simulink library "sm_mining_loader_lib"  (R2026a)
settings: Solver=VariableStepAuto
undefined symbols (not defined in the file): FL, FR, Init, LL, LR, Maneuver, minMachParams, motGradParams, RL, RR, simscape, SL, SR, T, X, Y, Z
libraries: sm_lib x130, nesl_utility x77, fl_lib x36, sdl_lib x11, simulink x4, $bdroot x3, sm_vehicle_utilities_lib x2, simulink_extras x2, statsLibrary x1, grid_element x1, Maneuver_Get_Pose x1
(part 2 of 6)

== system sm_mining_loader_lib/Mining Loader/Vehicle/Camera Frames F ==
  Cam Ref Ctr : sm_lib/Frames and Transforms/Reference Frame
  Cam Ref FL : sm_lib/Frames and Transforms/Reference Frame
  Cam Ref FR : sm_lib/Frames and Transforms/Reference Frame
  Cam Ref Left : sm_lib/Frames and Transforms/Reference Frame
  Cam Ref Right : sm_lib/Frames and Transforms/Reference Frame
  Cam Ref Top Down : sm_lib/Frames and Transforms/Reference Frame
  Cam Ref Top Rear Fwd : sm_lib/Frames and Transforms/Reference Frame
  Transform Ctr : sm_lib/Frames and Transforms/Rigid Transform  RotationMethod=None  FollAlignAxisA=+X  BaseAlignAxisA=+Y  FollAlignAxisB=+Y  BaseAlignAxisB=+Z  RotationStandardAxis=+Z  RotationAngle=0  RotationAngleUnits=deg  RotationArbitraryAxis=[0 0 1]  RotationSequenceAxes=FollowerAxes  RotationSequence=XYX  RotationSequenceAngles=[0 0 0]  RotationSequenceAnglesUnits=deg  RotationMatrix=[1 0 0;0 1 0;0 0 1]  Quaternion=[1 0 0 0]  TranslationMethod=StandardAxis  TranslationCartesianOffset=[0 0 0]  TranslationCartesianOffsetUnits=m  TranslationStandardAxis=+Z  TranslationStandardOffset=2  TranslationStandardOffsetUnits=m  TranslationROffset=0  TranslationROffsetUnits=m  TranslationThetaOffset=0  TranslationThetaOffsetUnits=deg  TranslationZOffset=0  TranslationZOffsetUnits=m
  Transform FL : sm_lib/Frames and Transforms/Rigid Transform  RotationMethod=None  FollAlignAxisA=+X  BaseAlignAxisA=+Y  FollAlignAxisB=+Y  BaseAlignAxisB=+Z  RotationStandardAxis=+Z  RotationAngle=0  RotationAngleUnits=deg  RotationArbitraryAxis=[0 0 1]  RotationSequenceAxes=FollowerAxes  RotationSequence=XYX  RotationSequenceAngles=[0 0 0]  RotationSequenceAnglesUnits=deg  RotationMatrix=[1 0 0;0 1 0;0 0 1]  Quaternion=[1 0 0 0]  TranslationMethod=Cartesian  TranslationCartesianOffset=[9 5 2]  TranslationCartesianOffsetUnits=m  TranslationStandardAxis=+Z  TranslationStandardOffset=2  TranslationStandardOffsetUnits=m  TranslationROffset=0  TranslationROffsetUnits=m  TranslationThetaOffset=0  TranslationThetaOffsetUnits=deg  TranslationZOffset=0  TranslationZOffsetUnits=m
  Transform FR : sm_lib/Frames and Transforms/Rigid Transform  RotationMethod=None  FollAlignAxisA=+X  BaseAlignAxisA=+Y  FollAlignAxisB=+Y  BaseAlignAxisB=+Z  RotationStandardAxis=+Z  RotationAngle=0  RotationAngleUnits=deg  RotationArbitraryAxis=[0 0 1]  RotationSequenceAxes=FollowerAxes  RotationSequence=XYX  RotationSequenceAngles=[0 0 0]  RotationSequenceAnglesUnits=deg  RotationMatrix=[1 0 0;0 1 0;0 0 1]  Quaternion=[1 0 0 0]  TranslationMethod=Cartesian  TranslationCartesianOffset=[9 -5 2]  TranslationCartesianOffsetUnits=m  TranslationStandardAxis=+Z  TranslationStandardOffset=2  TranslationStandardOffsetUnits=m  TranslationROffset=0  TranslationROffsetUnits=m  TranslationThetaOffset=0  TranslationThetaOffsetUnits=deg  TranslationZOffset=0  TranslationZOffsetUnits=m
  Transform Left : sm_lib/Frames and Transforms/Rigid Transform  RotationMethod=None  FollAlignAxisA=+X  BaseAlignAxisA=+Y  FollAlignAxisB=+Y  BaseAlignAxisB=+Z  RotationStandardAxis=+Z  RotationAngle=0  RotationAngleUnits=deg  RotationArbitraryAxis=[0 0 1]  RotationSequenceAxes=FollowerAxes  RotationSequence=XYX  RotationSequenceAngles=[0 0 0]  RotationSequenceAnglesUnits=deg  RotationMatrix=[1 0 0;0 1 0;0 0 1]  Quaternion=[1 0 0 0]  TranslationMethod=Cartesian  TranslationCartesianOffset=[-2 -9 0]  TranslationCartesianOffsetUnits=m  TranslationStandardAxis=+Z  TranslationStandardOffset=2  TranslationStandardOffsetUnits=m  TranslationROffset=0  TranslationROffsetUnits=m  TranslationThetaOffset=0  TranslationThetaOffsetUnits=deg  TranslationZOffset=0  TranslationZOffsetUnits=m
  Transform Right : sm_lib/Frames and Transforms/Rigid Transform  RotationMethod=None  FollAlignAxisA=+X  BaseAlignAxisA=+Y  FollAlignAxisB=+Y  BaseAlignAxisB=+Z  RotationStandardAxis=+Z  RotationAngle=0  RotationAngleUnits=deg  RotationArbitraryAxis=[0 0 1]  RotationSequenceAxes=FollowerAxes  RotationSequence=XYX  RotationSequenceAngles=[0 0 0]  RotationSequenceAnglesUnits=deg  RotationMatrix=[1 0 0;0 1 0;0 0 1]  Quaternion=[1 0 0 0]  TranslationMethod=Cartesian  TranslationCartesianOffset=[-2 9 0]  TranslationCartesianOffsetUnits=m  TranslationStandardAxis=+Z  TranslationStandardOffset=2  TranslationStandardOffsetUnits=m  TranslationROffset=0  TranslationROffsetUnits=m  TranslationThetaOffset=0  TranslationThetaOffsetUnits=deg  TranslationZOffset=0  TranslationZOffsetUnits=m
  Transform Top : sm_lib/Frames and Transforms/Rigid Transform  RotationMethod=None  FollAlignAxisA=+X  BaseAlignAxisA=+Y  FollAlignAxisB=+Y  BaseAlignAxisB=+Z  RotationStandardAxis=+Z  RotationAngle=0  RotationAngleUnits=deg  RotationArbitraryAxis=[0 0 1]  RotationSequenceAxes=FollowerAxes  RotationSequence=XYX  RotationSequenceAngles=[0 0 0]  RotationSequenceAnglesUnits=deg  RotationMatrix=[1 0 0;0 1 0;0 0 1]  Quaternion=[1 0 0 0]  TranslationMethod=Cartesian  TranslationCartesianOffset=[-2 0 13]  TranslationCartesianOffsetUnits=m  TranslationStandardAxis=+Z  TranslationStandardOffset=10  TranslationStandardOffsetUnits=m  TranslationROffset=0  TranslationROffsetUnits=m  TranslationThetaOffset=0  TranslationThetaOffsetUnits=deg  TranslationZOffset=0  TranslationZOffsetUnits=m
  Transform Top Rear Fwd : sm_lib/Frames and Transforms/Rigid Transform  RotationMethod=None  FollAlignAxisA=+X  BaseAlignAxisA=+Y  FollAlignAxisB=+Y  BaseAlignAxisB=+Z  RotationStandardAxis=+Z  RotationAngle=0  RotationAngleUnits=deg  RotationArbitraryAxis=[0 0 1]  RotationSequenceAxes=FollowerAxes  RotationSequence=XYX  RotationSequenceAngles=[0 0 0]  RotationSequenceAnglesUnits=deg  RotationMatrix=[1 0 0;0 1 0;0 0 1]  Quaternion=[1 0 0 0]  TranslationMethod=Cartesian  TranslationCartesianOffset=[-4 0 1]  TranslationCartesianOffsetUnits=m  TranslationStandardAxis=+Z  TranslationStandardOffset=2  TranslationStandardOffsetUnits=m  TranslationROffset=0  TranslationROffsetUnits=m  TranslationThetaOffset=0  TranslationThetaOffsetUnits=deg  TranslationZOffset=0  TranslationZOffsetUnits=m
  R : PMIOPort  Side=Left
  connections:
  Cam Ref FL/RConn1 -- Transform FL/RConn1
  Cam Ref FR/RConn1 -- Transform FR/RConn1
  Transform Ctr/LConn1 -- R/RConn1
  Transform Top/LConn1 -- Transform Left/LConn1 -- Transform Right/LConn1 -- Cam Ref Ctr/RConn1 -- Transform FL/LConn1 -- Transform Top Rear Fwd/LConn1 -- Transform Ctr/RConn1 -- Transform FR/LConn1
  Cam Ref Right/RConn1 -- Transform Right/RConn1
  Cam Ref Left/RConn1 -- Transform Left/RConn1
  Cam Ref Top Down/RConn1 -- Transform Top/RConn1
  Cam Ref Top Rear Fwd/RConn1 -- Transform Top Rear Fwd/RConn1

== system sm_mining_loader_lib/Mining Loader/Vehicle/Camera Frames R ==
  Cam Ref Ctr : sm_lib/Frames and Transforms/Reference Frame
  Cam Ref LR : sm_lib/Frames and Transforms/Reference Frame
  Cam Ref Left : sm_lib/Frames and Transforms/Reference Frame
  Cam Ref RR : sm_lib/Frames and Transforms/Reference Frame
  Cam Ref Right : sm_lib/Frames and Transforms/Reference Frame
  Cam Ref Top Down : sm_lib/Frames and Transforms/Reference Frame
  Cam Ref Top Rear Fwd : sm_lib/Frames and Transforms/Reference Frame
  Transform Ctr : sm_lib/Frames and Transforms/Rigid Transform  RotationMethod=None  FollAlignAxisA=+X  BaseAlignAxisA=+Y  FollAlignAxisB=+Y  BaseAlignAxisB=+Z  RotationStandardAxis=+Z  RotationAngle=0  RotationAngleUnits=deg  RotationArbitraryAxis=[0 0 1]  RotationSequenceAxes=FollowerAxes  RotationSequence=XYX  RotationSequenceAngles=[0 0 0]  RotationSequenceAnglesUnits=deg  RotationMatrix=[1 0 0;0 1 0;0 0 1]  Quaternion=[1 0 0 0]  TranslationMethod=StandardAxis  TranslationCartesianOffset=[0 0 0]  TranslationCartesianOffsetUnits=m  TranslationStandardAxis=+Z  TranslationStandardOffset=2  TranslationStandardOffsetUnits=m  TranslationROffset=0  TranslationROffsetUnits=m  TranslationThetaOffset=0  TranslationThetaOffsetUnits=deg  TranslationZOffset=0  TranslationZOffsetUnits=m
  Transform LR : sm_lib/Frames and Transforms/Rigid Transform  RotationMethod=None  FollAlignAxisA=+X  BaseAlignAxisA=+Y  FollAlignAxisB=+Y  BaseAlignAxisB=+Z  RotationStandardAxis=+Z  RotationAngle=0  RotationAngleUnits=deg  RotationArbitraryAxis=[0 0 1]  RotationSequenceAxes=FollowerAxes  RotationSequence=XYX  RotationSequenceAngles=[0 0 0]  RotationSequenceAnglesUnits=deg  RotationMatrix=[1 0 0;0 1 0;0 0 1]  Quaternion=[1 0 0 0]  TranslationMethod=Cartesian  TranslationCartesianOffset=[-8 -5 2]  TranslationCartesianOffsetUnits=m  TranslationStandardAxis=+Z  TranslationStandardOffset=2  TranslationStandardOffsetUnits=m  TranslationROffset=0  TranslationROffsetUnits=m  TranslationThetaOffset=0  TranslationThetaOffsetUnits=deg  TranslationZOffset=0  TranslationZOffsetUnits=m
  Transform Left : sm_lib/Frames and Transforms/Rigid Transform  RotationMethod=None  FollAlignAxisA=+X  BaseAlignAxisA=+Y  FollAlignAxisB=+Y  BaseAlignAxisB=+Z  RotationStandardAxis=+Z  RotationAngle=0  RotationAngleUnits=deg  RotationArbitraryAxis=[0 0 1]  RotationSequenceAxes=FollowerAxes  RotationSequence=XYX  RotationSequenceAngles=[0 0 0]  RotationSequenceAnglesUnits=deg  RotationMatrix=[1 0 0;0 1 0;0 0 1]  Quaternion=[1 0 0 0]  TranslationMethod=Cartesian  TranslationCartesianOffset=[1.85 -9 0]  TranslationCartesianOffsetUnits=m  TranslationStandardAxis=+Z  TranslationStandardOffset=2  TranslationStandardOffsetUnits=m  TranslationROffset=0  TranslationROffsetUnits=m  TranslationThetaOffset=0  TranslationThetaOffsetUnits=deg  TranslationZOffset=0  TranslationZOffsetUnits=m
  Transform RR : sm_lib/Frames and Transforms/Rigid Transform  RotationMethod=None  FollAlignAxisA=+X  BaseAlignAxisA=+Y  FollAlignAxisB=+Y  BaseAlignAxisB=+Z  RotationStandardAxis=+Z  RotationAngle=0  RotationAngleUnits=deg  RotationArbitraryAxis=[0 0 1]  RotationSequenceAxes=FollowerAxes  RotationSequence=XYX  RotationSequenceAngles=[0 0 0]  RotationSequenceAnglesUnits=deg  RotationMatrix=[1 0 0;0 1 0;0 0 1]  Quaternion=[1 0 0 0]  TranslationMethod=Cartesian  TranslationCartesianOffset=[-8 5 2]  TranslationCartesianOffsetUnits=m  TranslationStandardAxis=+Z  TranslationStandardOffset=2  TranslationStandardOffsetUnits=m  TranslationROffset=0  TranslationROffsetUnits=m  TranslationThetaOffset=0  TranslationThetaOffsetUnits=deg  TranslationZOffset=0  TranslationZOffsetUnits=m
  Transform Right : sm_lib/Frames and Transforms/Rigid Transform  RotationMethod=None  FollAlignAxisA=+X  BaseAlignAxisA=+Y  FollAlignAxisB=+Y  BaseAlignAxisB=+Z  RotationStandardAxis=+Z  RotationAngle=0  RotationAngleUnits=deg  RotationArbitraryAxis=[0 0 1]  RotationSequenceAxes=FollowerAxes  RotationSequence=XYX  RotationSequenceAngles=[0 0 0]  RotationSequenceAnglesUnits=deg  RotationMatrix=[1 0 0;0 1 0;0 0 1]  Quaternion=[1 0 0 0]  TranslationMethod=Cartesian  TranslationCartesianOffset=[1.85 9 0]  TranslationCartesianOffsetUnits=m  TranslationStandardAxis=+Z  TranslationStandardOffset=2  TranslationStandardOffsetUnits=m  TranslationROffset=0  TranslationROffsetUnits=m  TranslationThetaOffset=0  TranslationThetaOffsetUnits=deg  TranslationZOffset=0  TranslationZOffsetUnits=m
  Transform Top : sm_lib/Frames and Transforms/Rigid Transform  RotationMethod=None  FollAlignAxisA=+X  BaseAlignAxisA=+Y  FollAlignAxisB=+Y  BaseAlignAxisB=+Z  RotationStandardAxis=+Z  RotationAngle=0  RotationAngleUnits=deg  RotationArbitraryAxis=[0 0 1]  RotationSequenceAxes=FollowerAxes  RotationSequence=XYX  RotationSequenceAngles=[0 0 0]  RotationSequenceAnglesUnits=deg  RotationMatrix=[1 0 0;0 1 0;0 0 1]  Quaternion=[1 0 0 0]  TranslationMethod=Cartesian  TranslationCartesianOffset=[1.85 0 13]  TranslationCartesianOffsetUnits=m  TranslationStandardAxis=+Z  TranslationStandardOffset=10  TranslationStandardOffsetUnits=m  TranslationROffset=0  TranslationROffsetUnits=m  TranslationThetaOffset=0  TranslationThetaOffsetUnits=deg  TranslationZOffset=0  TranslationZOffsetUnits=m
  Transform Top Rear Fwd : sm_lib/Frames and Transforms/Rigid Transform  RotationMethod=None  FollAlignAxisA=+X  BaseAlignAxisA=+Y  FollAlignAxisB=+Y  BaseAlignAxisB=+Z  RotationStandardAxis=+Z  RotationAngle=0  RotationAngleUnits=deg  RotationArbitraryAxis=[0 0 1]  RotationSequenceAxes=FollowerAxes  RotationSequence=XYX  RotationSequenceAngles=[0 0 0]  RotationSequenceAnglesUnits=deg  RotationMatrix=[1 0 0;0 1 0;0 0 1]  Quaternion=[1 0 0 0]  TranslationMethod=Cartesian  TranslationCartesianOffset=[-0.15 0 1]  TranslationCartesianOffsetUnits=m  TranslationStandardAxis=+Z  TranslationStandardOffset=2  TranslationStandardOffsetUnits=m  TranslationROffset=0  TranslationROffsetUnits=m  TranslationThetaOffset=0  TranslationThetaOffsetUnits=deg  TranslationZOffset=0  TranslationZOffsetUnits=m
  R : PMIOPort  Side=Left
  connections:
  Transform Top Rear Fwd/LConn1 -- Transform Ctr/RConn1 -- Transform RR/LConn1 -- Transform LR/LConn1 -- Cam Ref Ctr/RConn1 -- Transform Right/LConn1 -- Transform Top/LConn1 -- Transform Left/LConn1
  Transform Ctr/LConn1 -- R/RConn1
  Cam Ref LR/RConn1 -- Transform LR/RConn1
  Cam Ref RR/RConn1 -- Transform RR/RConn1
  Cam Ref Top Rear Fwd/RConn1 -- Transform Top Rear Fwd/RConn1
  Cam Ref Right/RConn1 -- Transform Right/RConn1
  Cam Ref Left/RConn1 -- Transform Left/RConn1
  Cam Ref Top Down/RConn1 -- Transform Top/RConn1

== system sm_mining_loader_lib/Mining Loader/Vehicle/Chassis ==
  Housing : Subsystem
      mask Display: image('sm_mining_loader_chassis_housing_IMAGE.png')
  Revolute Whl RL : Subsystem
  Revolute Whl RR : Subsystem
  Whl RL : Subsystem
      mask Display: image('sm_mining_loader_wheel_IMAGE.png')
  Whl RR : Subsystem
      mask Display: image('sm_mining_loader_wheel_IMAGE.png')
  Ref : PMIOPort  Side=Left
  Ground : PMIOPort  Port=2  Side=Left
  Hinge : PMIOPort  Port=3  Side=Right
  StrL : PMIOPort  Port=4  Side=Right
  StrR : PMIOPort  Port=5  Side=Right
  LR : PMIOPort  Port=6  Side=Right
  RR : PMIOPort  Port=7  Side=Right
  Out Bus Element : Outport  PortName=m  Element=WhlRL
  Out Bus Element1 : Outport  PortName=m  Element=WhlRR
  Out Bus Element2 : Outport  PortName=m  Element=TireRL
  Out Bus Element3 : Outport  PortName=m  Element=TireRR
  wires:
  Revolute Whl RR/1(m) -> Out Bus Element1/1
  Revolute Whl RL/1(m) -> Out Bus Element/1
  Whl RL/1(m) -> Out Bus Element2/1
  Whl RR/1(m) -> Out Bus Element3/1
  connections:
  Ground/RConn1 -- Whl RL/RConn1 -- Whl RR/RConn1
  RR/RConn1 -- Revolute Whl RR/LConn1
  Whl RR/LConn1 -- Revolute Whl RR/LConn2
  Revolute Whl RL/LConn1 -- LR/RConn1
  Whl RL/LConn1 -- Revolute Whl RL/LConn2
  Housing/LConn3 -- Ref/RConn1
  StrR/RConn1 -- Housing/LConn4
  StrL/RConn1 -- Housing/LConn1
  Housing/LConn2 -- Hinge/RConn1
  Revolute Whl RL/RConn1 -- Housing/RConn1
  Revolute Whl RR/RConn1 -- Housing/RConn2

== system sm_mining_loader_lib/Mining Loader/Vehicle/Frame ==
  Body Sensor : sm_vehicle_utilities_lib/Body Sensor  offset_body_sensor=[0 0 0]
  Housing : Subsystem
      settings: PortSchema="{\"entries\":[{\"content\":{\"sides\":[{\"content\":{\"connectorIds\":[\"LConn1\",\"LConn2\",\"LConn3\",\"LConn4\"]},\"type\":\"ConnectorPlacement.EquallySpacedRectSide\",\"uuid\":\"fdb8be9a-7bb9-4005-a3a7-01384b0c122c\"},{\"content\":{\"connectorIds\":[\"RConn1\",\"RConn2\",\"RConn3\",\"RConn4\"],\"side\":\"RIGHT\"},\"type\":\"ConnectorPlacement.EquallySpacedRectSide\",\"uuid\":\"1ae00c9e-27b3-4807-843a-3ea8306620e4\"},{\"content\":{\"side\":\"TOP\"},\"type\":\"ConnectorPlacement.EquallySpacedRectSide\",\"uuid\":\"0a0d877e-6f75-4a01-a1db-7b7603a65aa1\"},{\"content\":{\"connectorIds\":[\"RConn5\"],\"side\":\"BOTTOM\"},\"type\":\"ConnectorPlacement.EquallySpacedRectSide\",\"uuid\":\"108f17e2-93b2-4dab-87d6-e955d5a596de\"}]},\"type\":\"ConnectorPlacement.EquallySpacedConnector\",\"uuid\":\"ae288347-5c86-4488-a1cc-f8f672d51556\"}],\"packageUris\":[\"http://schema.mathworks.com/mf0/Connector/R2020b\"],\"version\":\"1.0\"}"
      mask Display: image('sm_mining_loader_frame_housing_IMAGE.png')
  Revolute Whl FL : Subsystem
  Revolute Whl FR : Subsystem
  Whl FL : Subsystem
      mask Display: image('sm_mining_loader_wheel_IMAGE.png')
  Whl FR : Subsystem
      mask Display: image('sm_mining_loader_wheel_IMAGE.png')
  Hinge : PMIOPort  Side=Left
  StrL : PMIOPort  Port=2  Side=Left
  StrR : PMIOPort  Port=3  Side=Left
  FR : PMIOPort  Port=4  Side=Left
  FL : PMIOPort  Port=5  Side=Left
  LiftL : PMIOPort  Port=6  Side=Right
  LiftR : PMIOPort  Port=7  Side=Right
  Boom : PMIOPort  Port=8  Side=Right
  Ground : PMIOPort  Port=9  Side=Right
  Ref : PMIOPort  Port=10  Side=Right
  Out Bus Element : Outport  PortName=m  Element=WhlFL
  Out Bus Element1 : Outport  PortName=m  Element=WhlFR
  Out Bus Element2 : Outport  PortName=m  Element=Body
  Out Bus Element3 : Outport  PortName=m  Element=TireFL
  Out Bus Element4 : Outport  PortName=m  Element=TireFR
  wires:
  Revolute Whl FL/1(m) -> Out Bus Element/1
  Revolute Whl FR/1(m) -> Out Bus Element1/1
  Body Sensor/1 -> Out Bus Element2/1
  Whl FL/1(m) -> Out Bus Element3/1
  Whl FR/1(m) -> Out Bus Element4/1
  connections:
  Ground/RConn1 -- Whl FL/RConn1 -- Whl FR/RConn1
  FL/RConn1 -- Revolute Whl FL/LConn1
  Whl FL/LConn1 -- Revolute Whl FL/LConn2
  FR/RConn1 -- Revolute Whl FR/LConn1
  Whl FR/LConn1 -- Revolute Whl FR/LConn2
  Body Sensor/LConn1 -- Housing/LConn4 -- Ref/RConn1
  Revolute Whl FL/RConn1 -- Housing/LConn1
  Revolute Whl FR/RConn1 -- Housing/RConn1
  StrL/RConn1 -- Housing/LConn2
  Housing/RConn5 -- Hinge/RConn1
  StrR/RConn1 -- Housing/RConn2
  Boom/RConn1 -- Housing/RConn4
  LiftL/RConn1 -- Housing/LConn3
  Housing/RConn3 -- LiftR/RConn1

== system sm_mining_loader_lib/Mining Loader/Vehicle/Implement ==
  qBucket : Inport
  qBoom : Inport  Port=2
  In Bus Element : Inport  Port=3  PortName=Load
  Boom : Subsystem
      mask Display: image('sm_mining_loader_impl_boom_IMAGE.png')
  Lift Actuators : Subsystem  mask{popup_lift_actuation=Hinge Motion}
      mask prompts: popup_lift_actuation "Lift Actuation"
      mask init:
      | bh = gcb;
      | actSetting = get_param(bh,'popup_lift_actuation');
      | switch actSetting
      |     case('Hinge Motion')
      |         labelStr = 'Hinge';
      |     case('Left Cylinder Motion')
      |         labelStr = 'Extension_L';
      |     case('Cylinder Actuation')
      |         labelStr = 'Actuation';
      | end
      | set_param([bh '/Actuation'],'LabelModeActiveChoice',labelStr)
      settings: AttributesFormatString=%<popup_lift_actuation>
      mask TypeOptions popup_lift_actuation: Hinge Motion | Left Cylinder Motion | Cylinder Actuation
      mask Display:
      | bh = gcb;
      | 
      | actSetting = get_param(bh,'popup_lift_actuation');
      | 
      | switch actSetting
      |     case('Hinge Motion')
      |         imageStr = 'sm_mining_loader_lift_hinge_motion_IMAGE.png';
      |     case('Left Cylinder Motion')
      |         imageStr = 'sm_mining_loader_lift_cyl_motion_IMAGE.png';
      |     case('Cylinder Actuation')
      |         imageStr = 'sm_mining_loader_lift_cyl_actuation_IMAGE.png';
      | end
      | image(imageStr)
  Linkage : Subsystem
      mask Display: image('sm_mining_loader_impl_bucket_IMAGE.png')
  Tilt Actuator : Subsystem  mask{popup_tilt_actuation=Hinge Motion}
      mask prompts: popup_tilt_actuation "Tilt Actuation"
      mask init:
      | bh = gcb;
      | actSetting = get_param(bh,'popup_tilt_actuation');
      | switch actSetting
      |     case('Hinge Motion')
      |         labelStr = 'Hinge';
      |     case('Cylinder Motion')
      |         labelStr = 'Extension';
      |     case('Cylinder Actuation')
      |         labelStr = 'Actuation';
      | end
      | set_param([bh '/Actuation'],'LabelModeActiveChoice',labelStr)
      settings: AttributesFormatString=%<popup_tilt_actuation>
      mask TypeOptions popup_tilt_actuation: Hinge Motion | Cylinder Motion | Cylinder Actuation
      mask Display:
      | bh = gcb;
      | 
      | actSetting = get_param(bh,'popup_tilt_actuation');
      | 
      | switch actSetting
      |     case('Hinge Motion')
      |         imageStr = 'sm_mining_loader_tilt_hinge_motion_IMAGE.png';
      |     case('Cylinder Motion')
      |         imageStr = 'sm_mining_loader_tilt_cyl_motion_IMAGE.png';
      |     case('Cylinder Actuation')
      |         imageStr = 'sm_mining_loader_tilt_cyl_actuation_IMAGE.png';
      | end
      | image(imageStr)
  LIftL : PMIOPort  Side=Left
  LiftR : PMIOPort  Port=2  Side=Left
  Frame : PMIOPort  Port=3  Side=Left
  LL : PMIOPort  Port=4  Side=Right
  LR : PMIOPort  Port=5  Side=Right
  T : PMIOPort  Port=6  Side=Right
  Lift : Outport
  Tilt : Outport  Port=2
  Bucket : Outport  Port=3
  wires:
  qBucket/1 -> Tilt Actuator/1(qBucket)
  qBoom/1 -> Lift Actuators/1(qBoom)
  Lift Actuators/1(m) -> Lift/1
  Tilt Actuator/1(m) -> Tilt/1
  Linkage/1(m) -> Bucket/1
  In Bus Element/1 -> Linkage/1(Load)
  connections:
  Lift Actuators/RConn3 -- Boom/LConn2
  Lift Actuators/RConn2 -- Boom/LConn1
  Boom/LConn3 -- Lift Actuators/RConn4
  Lift Actuators/LConn3 -- LiftR/RConn1
  Lift Actuators/LConn4 -- Frame/RConn1
  Lift Actuators/LConn2 -- LIftL/RConn1
  LR/RConn1 -- Lift Actuators/RConn1
  LL/RConn1 -- Lift Actuators/LConn1
  T/RConn1 -- Tilt Actuator/LConn1
  Boom/RConn2 -- Tilt Actuator/LConn3
  Linkage/LConn2 -- Tilt Actuator/RConn3
  Linkage/LConn3 -- Boom/RConn3
  Boom/RConn1 -- Tilt Actuator/LConn2
  Tilt Actuator/RConn2 -- Linkage/LConn1

== system sm_mining_loader_lib/Mining Loader/Vehicle/Steer ==
  qStr : Inport
  Actuation : Subsystem  Variant=on  VariantControlMode=label  LabelModeActiveChoice=Hinge
      settings: AttributesFormatString=%<LabelModeActiveChoice>
  Cylinder Left : sm_lib/Body Elements/File Solid  ExtGeomFileName=SteerCylinder.step  UnitType=FromFile  ExtGeomFileUnits=m  StepReaderType=HEX  ExportConvexHullGeometry=off  InertiaType=CalculateFromGeometry  BasedOnType=Mass  Density=1000  DensityUnits=kg/m^3  Mass=minMachParams.steerCyl.mass  MassUnits=kg  CenterOfMass=[0 0 0]  CenterOfMassUnits=m  MomentsOfInertia=[1 1 1]  MomentsOfInertiaUnits=kg*m^2  ProductsOfInertia=[0 0 0]  ProductsOfInertiaUnits=kg*m^2  GraphicType=FromGeometry  MarkerShape=Sphere  MarkerSize=10  GraphicVisPropType=SimpleVisualProperties  GraphicDiffuseColor=[0.1 0.1 0.1]  GraphicOpacity=1  GraphicSpecularColor=[0.5 0.5 0.5 1.0]  GraphicAmbientColor=[0.15 0.15 0.15 1.0]  GraphicEmissiveColor=[0.0 0.0 0.0 1.0]  GraphicShininess=75  DoExposeReferenceFrame=off  SerializedFrames=<Frames><Frame><Id>Frame1</Id><Value><Name>ToFrontChassis</Name><Origin><Source>GeometricFeature</Source><FeatureName>circular curve 12</FeatureName></Origin><PrimaryAxis><DefinedDirection>+Z</DefinedDirection><Source>ReferenceFrame</Source><SourceDirection>+Z</SourceDirection><FeatureName></FeatureName></PrimaryAxis><SecondaryAxis><DefinedDirection>+X</DefinedDirection><Source>ReferenceFrame</Source><SourceDirection>+X</SourceDirection><FeatureName></FeatureName></SecondaryAxis></Value></Frame><Frame><Id>Frame2</Id><Value><Name>ToSteerRod</Name><Origin><Source>GeometricFeature</Source><FeatureName>planar surface 2</FeatureName></Origin><PrimaryAxis><DefinedDirection>+Z</DefinedDirection><Source>ReferenceFrame</Source><SourceDirection>-Y</SourceDirection><FeatureName></FeatureName></PrimaryAxis><SecondaryAxis><DefinedDirection>+X</DefinedDirection><Source>ReferenceFrame</Source><SourceDirection>+X</SourceDirection><FeatureName></FeatureName></SecondaryAxis></Value></Frame></Frames>
  Cylinder Right : sm_lib/Body Elements/File Solid  ExtGeomFileName=SteerCylinder.step  UnitType=FromFile  ExtGeomFileUnits=m  StepReaderType=HEX  ExportConvexHullGeometry=off  InertiaType=CalculateFromGeometry  BasedOnType=Mass  Density=1000  DensityUnits=kg/m^3  Mass=minMachParams.steerCyl.mass  MassUnits=kg  CenterOfMass=[0 0 0]  CenterOfMassUnits=m  MomentsOfInertia=[1 1 1]  MomentsOfInertiaUnits=kg*m^2  ProductsOfInertia=[0 0 0]  ProductsOfInertiaUnits=kg*m^2  GraphicType=FromGeometry  MarkerShape=Sphere  MarkerSize=10  GraphicVisPropType=SimpleVisualProperties  GraphicDiffuseColor=[0.1 0.1 0.1]  GraphicOpacity=1  GraphicSpecularColor=[0.5 0.5 0.5 1.0]  GraphicAmbientColor=[0.15 0.15 0.15 1.0]  GraphicEmissiveColor=[0.0 0.0 0.0 1.0]  GraphicShininess=75  DoExposeReferenceFrame=off  SerializedFrames=<Frames><Frame><Id>Frame1</Id><Value><Name>ToFrontChassis</Name><Origin><Source>GeometricFeature</Source><FeatureName>circular curve 12</FeatureName></Origin><PrimaryAxis><DefinedDirection>+Z</DefinedDirection><Source>ReferenceFrame</Source><SourceDirection>+Z</SourceDirection><FeatureName></FeatureName></PrimaryAxis><SecondaryAxis><DefinedDirection>+X</DefinedDirection><Source>ReferenceFrame</Source><SourceDirection>+X</SourceDirection><FeatureName></FeatureName></SecondaryAxis></Value></Frame><Frame><Id>Frame2</Id><Value><Name>ToSteerRod</Name><Origin><Source>GeometricFeature</Source><FeatureName>planar surface 2</FeatureName></Origin><PrimaryAxis><DefinedDirection>+Z</DefinedDirection><Source>ReferenceFrame</Source><SourceDirection>-Y</SourceDirection><FeatureName></FeatureName></PrimaryAxis><SecondaryAxis><DefinedDirection>+X</DefinedDirection><Source>ReferenceFrame</Source><SourceDirection>+X</SourceDirection><FeatureName></FeatureName></SecondaryAxis></Value></Frame></Frames>
  Revolute CylL : sm_lib/Joints/Revolute Joint  JointMode=Normal  CompositeWrenchDir=FollowerOnBase  CompositeWrenchFrame=BaseFrame  SenseConstraintForce=off  SenseConstraintTorque=off  SenseTotalForce=off  SenseTotalTorque=off  PositionTargetSpecify=off  PositionTargetPriority=High  PositionTargetValue=0  PositionTargetValueUnits=deg  VelocityTargetSpecify=off  VelocityTargetPriority=High  VelocityTargetValue=0  VelocityTargetValueUnits=deg/s  EquilibriumPosition=0  EquilibriumPositionUnits=deg  SpringStiffness=0  SpringStiffnessUnits=N*m/deg  DampingCoefficient=0  DampingCoefficientUnits=N*m/(deg/s)  LowerLimitSpecify=off  LowerLimitBound=-90  LowerLimitBoundUnits=deg  LowerLimitStiffness=1e4  LowerLimitStiffnessUnits=N*m/deg  LowerLimitDamping=10  LowerLimitDampingUnits=N*m/(deg/s)  LowerLimitTransitionRegionWidth=0.1  LowerLimitTransitionRegionWidthUnits=deg  UpperLimitSpecify=off  UpperLimitBound=90  UpperLimitBoundUnits=deg  UpperLimitStiffness=1e4  UpperLimitStiffnessUnits=N*m/deg  UpperLimitDamping=10  UpperLimitDampingUnits=N*m/(deg/s)  UpperLimitTransitionRegionWidth=0.1  UpperLimitTransitionRegionWidthUnits=deg  TorqueActuationMode=NoTorque  MotionActuationMode=ComputedMotion  SensePosition=off  SenseVelocity=off  SenseAcceleration=off  SenseTorqueForce=off  SenseLowerLimitTorqueForce=off  SenseUpperLimitTorqueForce=off
  Revolute CylR : sm_lib/Joints/Revolute Joint  JointMode=Normal  CompositeWrenchDir=FollowerOnBase  CompositeWrenchFrame=BaseFrame  SenseConstraintForce=off  SenseConstraintTorque=off  SenseTotalForce=off  SenseTotalTorque=off  PositionTargetSpecify=off  PositionTargetPriority=High  PositionTargetValue=0  PositionTargetValueUnits=deg  VelocityTargetSpecify=off  VelocityTargetPriority=High  VelocityTargetValue=0  VelocityTargetValueUnits=deg/s  EquilibriumPosition=0  EquilibriumPositionUnits=deg  SpringStiffness=0  SpringStiffnessUnits=N*m/deg  DampingCoefficient=0  DampingCoefficientUnits=N*m/(deg/s)  LowerLimitSpecify=off  LowerLimitBound=-90  LowerLimitBoundUnits=deg  LowerLimitStiffness=1e4  LowerLimitStiffnessUnits=N*m/deg  LowerLimitDamping=10  LowerLimitDampingUnits=N*m/(deg/s)  LowerLimitTransitionRegionWidth=0.1  LowerLimitTransitionRegionWidthUnits=deg  UpperLimitSpecify=off  UpperLimitBound=90  UpperLimitBoundUnits=deg  UpperLimitStiffness=1e4  UpperLimitStiffnessUnits=N*m/deg  UpperLimitDamping=10  UpperLimitDampingUnits=N*m/(deg/s)  UpperLimitTransitionRegionWidth=0.1  UpperLimitTransitionRegionWidthUnits=deg  TorqueActuationMode=NoTorque  MotionActuationMode=ComputedMotion  SensePosition=off  SenseVelocity=off  SenseAcceleration=off  SenseTorqueForce=off  SenseLowerLimitTorqueForce=off  SenseUpperLimitTorqueForce=off
  Revolute RodL : sm_lib/Joints/Revolute Joint  JointMode=Normal  CompositeWrenchDir=FollowerOnBase  CompositeWrenchFrame=BaseFrame  SenseConstraintForce=off  SenseConstraintTorque=off  SenseTotalForce=off  SenseTotalTorque=off  PositionTargetSpecify=off  PositionTargetPriority=High  PositionTargetValue=0  PositionTargetValueUnits=deg  VelocityTargetSpecify=off  VelocityTargetPriority=High  VelocityTargetValue=0  VelocityTargetValueUnits=deg/s  EquilibriumPosition=0  EquilibriumPositionUnits=deg  SpringStiffness=0  SpringStiffnessUnits=N*m/deg  DampingCoefficient=0  DampingCoefficientUnits=N*m/(deg/s)  LowerLimitSpecify=off  LowerLimitBound=-90  LowerLimitBoundUnits=deg  LowerLimitStiffness=1e4  LowerLimitStiffnessUnits=N*m/deg  LowerLimitDamping=10  LowerLimitDampingUnits=N*m/(deg/s)  LowerLimitTransitionRegionWidth=0.1  LowerLimitTransitionRegionWidthUnits=deg  UpperLimitSpecify=off  UpperLimitBound=90  UpperLimitBoundUnits=deg  UpperLimitStiffness=1e4  UpperLimitStiffnessUnits=N*m/deg  UpperLimitDamping=10  UpperLimitDampingUnits=N*m/(deg/s)  UpperLimitTransitionRegionWidth=0.1  UpperLimitTransitionRegionWidthUnits=deg  TorqueActuationMode=NoTorque  MotionActuationMode=ComputedMotion  SensePosition=off  SenseVelocity=off  SenseAcceleration=off  SenseTorqueForce=off  SenseLowerLimitTorqueForce=off  SenseUpperLimitTorqueForce=off
  Revolute RodR : sm_lib/Joints/Revolute Joint  JointMode=Normal  CompositeWrenchDir=FollowerOnBase  CompositeWrenchFrame=BaseFrame  SenseConstraintForce=off  SenseConstraintTorque=off  SenseTotalForce=off  SenseTotalTorque=off  PositionTargetSpecify=off  PositionTargetPriority=High  PositionTargetValue=0  PositionTargetValueUnits=deg  VelocityTargetSpecify=off  VelocityTargetPriority=High  VelocityTargetValue=0  VelocityTargetValueUnits=deg/s  EquilibriumPosition=0  EquilibriumPositionUnits=deg  SpringStiffness=0  SpringStiffnessUnits=N*m/deg  DampingCoefficient=0  DampingCoefficientUnits=N*m/(deg/s)  LowerLimitSpecify=off  LowerLimitBound=-90  LowerLimitBoundUnits=deg  LowerLimitStiffness=1e4  LowerLimitStiffnessUnits=N*m/deg  LowerLimitDamping=10  LowerLimitDampingUnits=N*m/(deg/s)  LowerLimitTransitionRegionWidth=0.1  LowerLimitTransitionRegionWidthUnits=deg  UpperLimitSpecify=off  UpperLimitBound=90  UpperLimitBoundUnits=deg  UpperLimitStiffness=1e4  UpperLimitStiffnessUnits=N*m/deg  UpperLimitDamping=10  UpperLimitDampingUnits=N*m/(deg/s)  UpperLimitTransitionRegionWidth=0.1  UpperLimitTransitionRegionWidthUnits=deg  TorqueActuationMode=NoTorque  MotionActuationMode=ComputedMotion  SensePosition=off  SenseVelocity=off  SenseAcceleration=off  SenseTorqueForce=off  SenseLowerLimitTorqueForce=off  SenseUpperLimitTorqueForce=off
  Rod Left : sm_lib/Body Elements/File Solid  ExtGeomFileName=SteerRod.step  UnitType=FromFile  ExtGeomFileUnits=m  StepReaderType=HEX  ExportConvexHullGeometry=off  InertiaType=CalculateFromGeometry  BasedOnType=Mass  Density=1000  DensityUnits=kg/m^3  Mass=minMachParams.steerRod.mass  MassUnits=kg  CenterOfMass=[0 0 0]  CenterOfMassUnits=m  MomentsOfInertia=[1 1 1]  MomentsOfInertiaUnits=kg*m^2  ProductsOfInertia=[0 0 0]  ProductsOfInertiaUnits=kg*m^2  GraphicType=FromGeometry  MarkerShape=Sphere  MarkerSize=10  GraphicVisPropType=SimpleVisualProperties  GraphicDiffuseColor=[0.8824 0.8824 0.8824]  GraphicOpacity=1  GraphicSpecularColor=[0.5 0.5 0.5 1.0]  GraphicAmbientColor=[0.15 0.15 0.15 1.0]  GraphicEmissiveColor=[0.0 0.0 0.0 1.0]  GraphicShininess=75  DoExposeReferenceFrame=off  SerializedFrames=<Frames><Frame><Id>Frame1</Id><Value><Name>ToSteerCyl</Name><Origin><Source>GeometricFeature</Source><FeatureName>planar surface 1</FeatureName></Origin><PrimaryAxis><DefinedDirection>+Z</DefinedDirection><Source>ReferenceFrame</Source><SourceDirection>-Y</SourceDirection><FeatureName></FeatureName></PrimaryAxis><SecondaryAxis><DefinedDirection>+X</DefinedDirection><Source>ReferenceFrame</Source><SourceDirection>+X</SourceDirection><FeatureName></FeatureName></SecondaryAxis></Value></Frame><Frame><Id>Frame2</Id><Value><Name>ToFrontFrame</Name><Origin><Source>GeometricFeature</Source><FeatureName>circular curve 10</FeatureName></Origin><PrimaryAxis><DefinedDirection>+Z</DefinedDirection><Source>ReferenceFrame</Source><SourceDirection>+Z</SourceDirection><FeatureName></FeatureName></PrimaryAxis><SecondaryAxis><DefinedDirection>+X</DefinedDirection><Source>ReferenceFrame</Source><SourceDirection>+X</SourceDirection><FeatureName></FeatureName></SecondaryAxis></Value></Frame></Frames>
  Rod Right : sm_lib/Body Elements/File Solid  ExtGeomFileName=SteerRod.step  UnitType=FromFile  ExtGeomFileUnits=m  StepReaderType=HEX  ExportConvexHullGeometry=off  InertiaType=CalculateFromGeometry  BasedOnType=Mass  Density=1000  DensityUnits=kg/m^3  Mass=minMachParams.steerRod.mass  MassUnits=kg  CenterOfMass=[0 0 0]  CenterOfMassUnits=m  MomentsOfInertia=[1 1 1]  MomentsOfInertiaUnits=kg*m^2  ProductsOfInertia=[0 0 0]  ProductsOfInertiaUnits=kg*m^2  GraphicType=FromGeometry  MarkerShape=Sphere  MarkerSize=10  GraphicVisPropType=SimpleVisualProperties  GraphicDiffuseColor=[0.8824 0.8824 0.8824]  GraphicOpacity=1  GraphicSpecularColor=[0.5 0.5 0.5 1.0]  GraphicAmbientColor=[0.15 0.15 0.15 1.0]  GraphicEmissiveColor=[0.0 0.0 0.0 1.0]  GraphicShininess=75  DoExposeReferenceFrame=off  SerializedFrames=<Frames><Frame><Id>Frame1</Id><Value><Name>ToSteerCyl</Name><Origin><Source>GeometricFeature</Source><FeatureName>planar surface 1</FeatureName></Origin><PrimaryAxis><DefinedDirection>+Z</DefinedDirection><Source>ReferenceFrame</Source><SourceDirection>-Y</SourceDirection><FeatureName></FeatureName></PrimaryAxis><SecondaryAxis><DefinedDirection>+X</DefinedDirection><Source>ReferenceFrame</Source><SourceDirection>+X</SourceDirection><FeatureName></FeatureName></SecondaryAxis></Value></Frame><Frame><Id>Frame2</Id><Value><Name>ToFrontFrame</Name><Origin><Source>GeometricFeature</Source><FeatureName>circular curve 10</FeatureName></Origin><PrimaryAxis><DefinedDirection>+Z</DefinedDirection><Source>ReferenceFrame</Source><SourceDirection>+Z</SourceDirection><FeatureName></FeatureName></PrimaryAxis><SecondaryAxis><DefinedDirection>+X</DefinedDirection><Source>ReferenceFrame</Source><SourceDirection>+X</SourceDirection><FeatureName></FeatureName></SecondaryAxis></Value></Frame></Frames>
  ActL : PMIOPort  Side=Left
  R : PMIOPort  Port=2  Side=Left
  CylL : PMIOPort  Port=3  Side=Left
  CylR : PMIOPort  Port=4  Side=Left
  ActR : PMIOPort  Port=5  Side=Right
  F : PMIOPort  Port=6  Side=Right
  RodL : PMIOPort  Port=7  Side=Right
  RodR : PMIOPort  Port=8  Side=Right
  m : Outport
  wires:
  qStr/1 -> Actuation/1(qStr)
  Actuation/1(m) -> m/1
  connections:
  R/RConn1 -- Actuation/LConn2
  Actuation/LConn3 -- Cylinder Left/RConn1
  F/RConn1 -- Actuation/RConn2
  Actuation/LConn4 -- Cylinder Right/RConn1
  Rod Left/LConn1 -- Actuation/RConn3
  Rod Right/LConn1 -- Actuation/RConn4
  Rod Left/RConn1 -- Revolute RodL/LConn1
  Revolute CylL/RConn1 -- Cylinder Left/LConn1
  Revolute CylR/RConn1 -- Cylinder Right/LConn1
  CylL/RConn1 -- Revolute CylL/LConn1
  RodL/RConn1 -- Revolute RodL/RConn1
  RodR/RConn1 -- Revolute RodR/RConn1
  Rod Right/RConn1 -- Revolute RodR/LConn1
  CylR/RConn1 -- Revolute CylR/LConn1
  ActL/RConn1 -- Actuation/LConn1
  ActR/RConn1 -- Actuation/RConn1

== system sm_mining_loader_lib/Mining Loader/Actuation/Lift/Position ==
  Cmd : Inport
  Meas : Inport  Port=2
  Terminator : Terminator
  Terminator1 : Terminator
  L : PMIOPort  Side=Right
  R : PMIOPort  Port=2  Side=Right
  wires:
  Cmd/1 -> Terminator/1
  Meas/1 -> Terminator1/1

== system sm_mining_loader_lib/Mining Loader/Actuation/Steer/Position ==
  Cmd : Inport
  Meas : Inport  Port=2
  Terminator : Terminator
  Terminator1 : Terminator
  L : PMIOPort  Side=Right
  R : PMIOPort  Port=2  Side=Right
  wires:
  Cmd/1 -> Terminator/1
  Meas/1 -> Terminator1/1

== system sm_mining_loader_lib/Mining Loader/Actuation/Tilt/Position ==
  Cmd : Inport
  Meas : Inport  Port=2
  Terminator : Terminator
  Terminator1 : Terminator
  R : PMIOPort  Side=Right
  wires:
  Cmd/1 -> Terminator/1
  Meas/1 -> Terminator1/1
